simulink subsystem "rss_BattPwrHiLvl1Dia"  (R2023a)
settings: Solver=VariableStepAuto  StartTime=0.0  StopTime=10.0  RelTol=1e-3
undefined symbols (not defined in the file): Cdbl_pwrElecPwrMaxVal, ENM_TYPE_FALT, Gu16_ctBattPwrHiLvl1ConfCnt_C, Gu16_ctBattPwrHiLvl1RcvyCnt_C, Gu16_pwrBattPwrHiLvl1ConfTrs_C
libraries: lib_debounce x1, lib_fault_definiteness x1
settings Model: Creator=xiaoqiang.yuan  LastModifiedBy=xiaoqiang.yuan

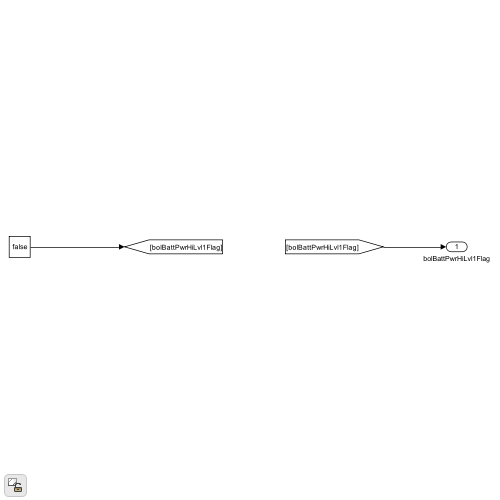
[thumbnail: Simulink's stored preview of the top-level diagram]
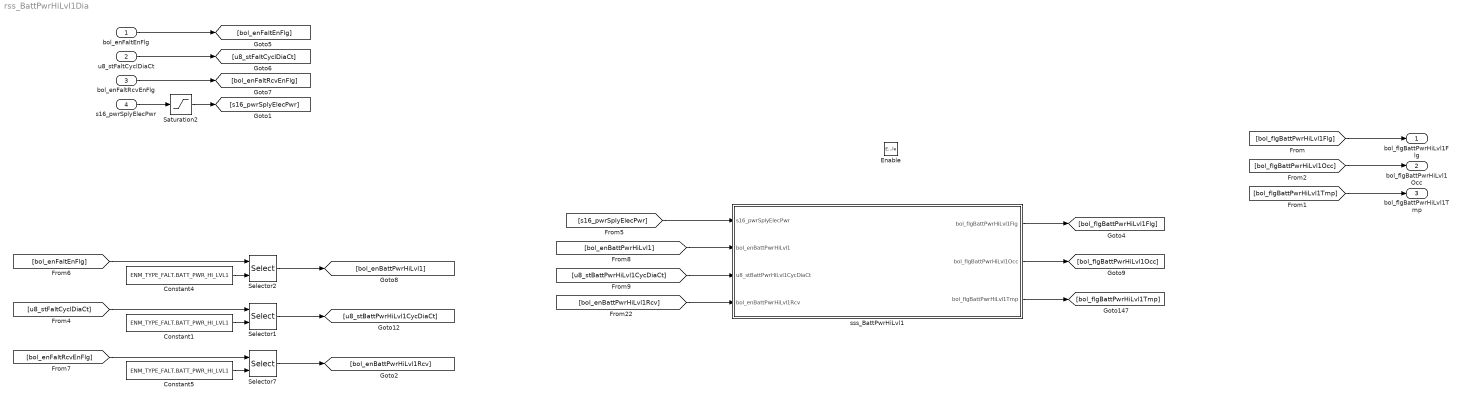
== system rss_BattPwrHiLvl1Dia ==
  bol_enFaltEnFlg : Inport  OutDataTypeStr=boolean
  u8_stFaltCyclDiaCt : Inport  Port=2  OutDataTypeStr=uint8
  bol_enFaltRcvEnFlg : Inport  Port=3  OutDataTypeStr=boolean
  s16_pwrSplyElecPwr : Inport  Port=4  OutDataTypeStr=dt_Standardize_s16p15b0
  Enable : EnablePort
  Constant1 : Constant  Value=ENM_TYPE_FALT.BATT_PWR_HI_LVL1
  Constant4 : Constant  Value=ENM_TYPE_FALT.BATT_PWR_HI_LVL1
  Constant5 : Constant  Value=ENM_TYPE_FALT.BATT_PWR_HI_LVL1
  Saturation2 : Saturate  UpperLimit=Cdbl_pwrElecPwrMaxVal  LowerLimit=-Cdbl_pwrElecPwrMaxVal
  Selector1 : Selector  IndexMode=Zero-based  InputPortWidth=Cdbl_numFaltDiaNum  IndexOptions=Index vector (port)  Indices=[1 3]  OutputSizes=1
  Selector2 : Selector  IndexMode=Zero-based  InputPortWidth=Cdbl_numFaltDiaNum  IndexOptions=Index vector (port)  Indices=[1 3]  OutputSizes=1
  Selector7 : Selector  IndexMode=Zero-based  InputPortWidth=Cdbl_numFaltDiaNum  IndexOptions=Index vector (port)  Indices=[1 3]  OutputSizes=1
  sss_BattPwrHiLvl1 : Subsystem
  bol_flgBattPwrHiLvl1Flg : Outport  OutDataTypeStr=boolean
  bol_flgBattPwrHiLvl1Occ : Outport  Port=2  OutDataTypeStr=boolean
  bol_flgBattPwrHiLvl1Tmp : Outport  Port=3  OutDataTypeStr=boolean
  wires:
  [bol_flgBattPwrHiLvl1Flg] -> bol_flgBattPwrHiLvl1Flg/1
  Selector1/1 -> [u8_stBattPwrHiLvl1CycDiaCt]
  [bol_enBattPwrHiLvl1] -> sss_BattPwrHiLvl1/2(bol_enBattPwrHiLvl1)
  s16_pwrSplyElecPwr/1 -> Saturation2/1
  sss_BattPwrHiLvl1/1(bol_flgBattPwrHiLvl1Flg) -> [bol_flgBattPwrHiLvl1Flg]
  bol_enFaltRcvEnFlg/1 -> [bol_enFaltRcvEnFlg]
  Saturation2/1 -> [s16_pwrSplyElecPwr]
  [bol_flgBattPwrHiLvl1Occ] -> bol_flgBattPwrHiLvl1Occ/1
  bol_enFaltEnFlg/1 -> [bol_enFaltEnFlg]
  [bol_enFaltEnFlg] -> Selector2/1
  [bol_enFaltRcvEnFlg] -> Selector7/1
  [u8_stBattPwrHiLvl1CycDiaCt] -> sss_BattPwrHiLvl1/3(u8_stBattPwrHiLvl1CycDiaCt)
  Selector2/1 -> [bol_enBattPwrHiLvl1]
  Selector7/1 -> [bol_enBattPwrHiLvl1Rcv]
  Constant4/1 -> Selector2/2
  sss_BattPwrHiLvl1/2(bol_flgBattPwrHiLvl1Occ) -> [bol_flgBattPwrHiLvl1Occ]
  [u8_stFaltCyclDiaCt] -> Selector1/1
  Constant1/1 -> Selector1/2
  [bol_enBattPwrHiLvl1Rcv] -> sss_BattPwrHiLvl1/4(bol_enBattPwrHiLvl1Rcv)
  [s16_pwrSplyElecPwr] -> sss_BattPwrHiLvl1/1(s16_pwrSplyElecPwr)
  Constant5/1 -> Selector7/2
  u8_stFaltCyclDiaCt/1 -> [u8_stFaltCyclDiaCt]
  [bol_flgBattPwrHiLvl1Tmp] -> bol_flgBattPwrHiLvl1Tmp/1
  sss_BattPwrHiLvl1/3(bol_flgBattPwrHiLvl1Tmp) -> [bol_flgBattPwrHiLvl1Tmp]

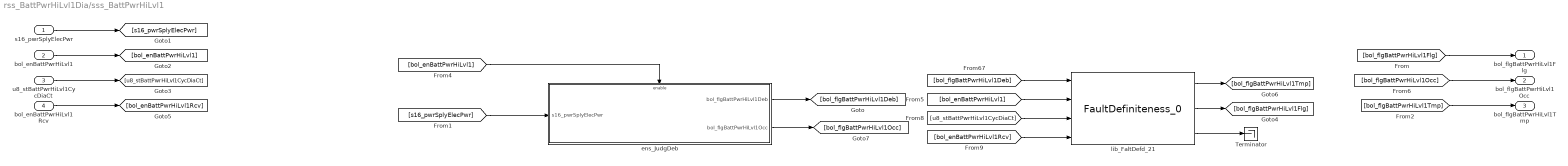
== system rss_BattPwrHiLvl1Dia/sss_BattPwrHiLvl1 ==
  s16_pwrSplyElecPwr : Inport
  bol_enBattPwrHiLvl1 : Inport  Port=2
  u8_stBattPwrHiLvl1CycDiaCt : Inport  Port=3
  bol_enBattPwrHiLvl1Rcv : Inport  Port=4
  Terminator : Terminator
  ens_JudgDeb : Subsystem
  lib_FaltDefd_21 : lib_fault_definiteness/FaultDefiniteness_0  lb_FaltWaitRecvCnt=Gu16_ctBattPwrHiLvl1ConfCnt_C
  bol_flgBattPwrHiLvl1Flg : Outport
  bol_flgBattPwrHiLvl1Occ : Outport  Port=2
  bol_flgBattPwrHiLvl1Tmp : Outport  Port=3
  wires:
  [bol_flgBattPwrHiLvl1Tmp] -> bol_flgBattPwrHiLvl1Tmp/1
  [bol_flgBattPwrHiLvl1Occ] -> bol_flgBattPwrHiLvl1Occ/1
  ens_JudgDeb/2(bol_flgBattPwrHiLvl1Occ) -> [bol_flgBattPwrHiLvl1Occ]
  lib_FaltDefd_21/1 -> [bol_flgBattPwrHiLvl1Tmp]
  lib_FaltDefd_21/2 -> [bol_flgBattPwrHiLvl1Flg]
  lib_FaltDefd_21/3 -> Terminator/1
  [bol_enBattPwrHiLvl1] -> ens_JudgDeb/Enable
  [s16_pwrSplyElecPwr] -> ens_JudgDeb/1(s16_pwrSplyElecPwr)
  ens_JudgDeb/1(bol_flgBattPwrHiLvl1Deb) -> [bol_flgBattPwrHiLvl1Deb]
  bol_enBattPwrHiLvl1Rcv/1 -> [bol_enBattPwrHiLvl1Rcv]
  u8_stBattPwrHiLvl1CycDiaCt/1 -> [u8_stBattPwrHiLvl1CycDiaCt]
  bol_enBattPwrHiLvl1/1 -> [bol_enBattPwrHiLvl1]
  [bol_flgBattPwrHiLvl1Flg] -> bol_flgBattPwrHiLvl1Flg/1
  s16_pwrSplyElecPwr/1 -> [s16_pwrSplyElecPwr]
  [bol_enBattPwrHiLvl1Rcv] -> lib_FaltDefd_21/4
  [u8_stBattPwrHiLvl1CycDiaCt] -> lib_FaltDefd_21/3
  [bol_enBattPwrHiLvl1] -> lib_FaltDefd_21/2
  [bol_flgBattPwrHiLvl1Deb] -> lib_FaltDefd_21/1

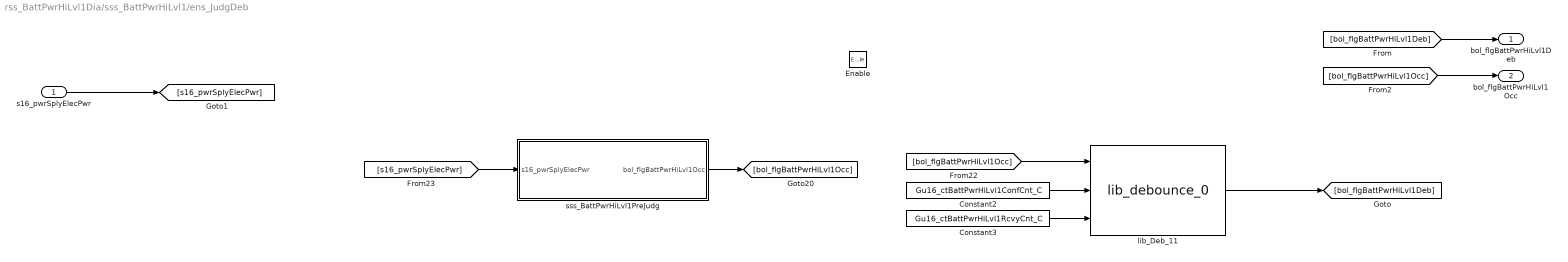
== system rss_BattPwrHiLvl1Dia/sss_BattPwrHiLvl1/ens_JudgDeb ==
  s16_pwrSplyElecPwr : Inport
  Enable : EnablePort
  Constant2 : Constant  Value=Gu16_ctBattPwrHiLvl1ConfCnt_C
  Constant3 : Constant  Value=Gu16_ctBattPwrHiLvl1RcvyCnt_C
  lib_Deb_11 : lib_debounce/lib_debounce_0
  sss_BattPwrHiLvl1PreJudg : Subsystem
  bol_flgBattPwrHiLvl1Deb : Outport
  bol_flgBattPwrHiLvl1Occ : Outport  Port=2
  wires:
  [bol_flgBattPwrHiLvl1Occ] -> bol_flgBattPwrHiLvl1Occ/1
  [s16_pwrSplyElecPwr] -> sss_BattPwrHiLvl1PreJudg/1(s16_pwrSplyElecPwr)
  s16_pwrSplyElecPwr/1 -> [s16_pwrSplyElecPwr]
  [bol_flgBattPwrHiLvl1Deb] -> bol_flgBattPwrHiLvl1Deb/1
  sss_BattPwrHiLvl1PreJudg/1(bol_flgBattPwrHiLvl1Occ) -> [bol_flgBattPwrHiLvl1Occ]
  Constant3/1 -> lib_Deb_11/3
  [bol_flgBattPwrHiLvl1Occ] -> lib_Deb_11/1
  lib_Deb_11/1 -> [bol_flgBattPwrHiLvl1Deb]
  Constant2/1 -> lib_Deb_11/2

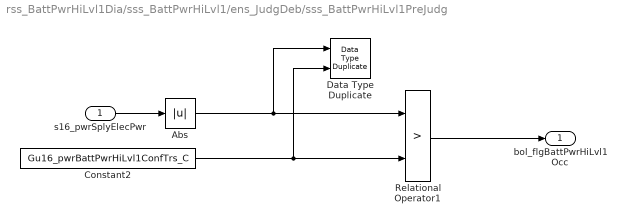
== system rss_BattPwrHiLvl1Dia/sss_BattPwrHiLvl1/ens_JudgDeb/sss_BattPwrHiLvl1PreJudg ==
  s16_pwrSplyElecPwr : Inport
  Abs : Abs  OutDataTypeStr=Inherit: Inherit via back propagation  SaturateOnIntegerOverflow=off
  Constant2 : Constant  Value=Gu16_pwrBattPwrHiLvl1ConfTrs_C
  Data Type Duplicate : DataTypeDuplicate
  Relational Operator1 : RelationalOperator  Operator=>  OutDataTypeStr=boolean  RndMeth=Simplest  InputSameDT=off
  bol_flgBattPwrHiLvl1Occ : Outport
  wires:
  Abs/1 -> Relational Operator1/1, Data Type Duplicate/1
  s16_pwrSplyElecPwr/1 -> Abs/1
  Relational Operator1/1 -> bol_flgBattPwrHiLvl1Occ/1
  Constant2/1 -> Relational Operator1/2, Data Type Duplicate/2
